simulink library "lib_HVESS"  (R2017a)
settings: Solver=VariableStepAuto  StartTime=0.0  StopTime=10.0  RelTol=1e-3
undefined symbols (not defined in the file): Atm_temp, bms_inletair_temp, bms_maxchargecurrent, bms_maxdischargecurrent, BMS_Notfallkuehlung, Cells, Chg, Em, ess, I_loss, mph2kph, R_0, R_1, SOC_bp, T_bp, tloop
libraries: fl_lib x13, simulink x9, nesl_utility x8, RollingAliveCounter x1
(part 2 of 2)

== stateflow chart lib_HVESS/ESS/Soft BMS/State Machine1/Startup_Shutdown_EPO_Sequence ==
  state BCM_ON
    state Default_Error_State
      en: BMS_Init_abgeschlossen=1;
      BMS_IstModus=5;
    state Standby
      en: BMS_Init_abgeschlossen=1;
      BMS_IstModus=0;
    state Normal_Driving
      en: NHM_BMS_Car_WakeUp=1;
      BMS_IstModus=1;
      BMS_Init_abgeschlossen=1;
      during: timer++;
    state Charging
      en:BMS_IstModus=4;
      BMS_Init_abgeschlossen =1;
      during: timer++;
    (default) -> Default_Error_State : [T_15&&T_30]
    Charging -> Default_Error_State [order 1] : [!T_30C]
    Normal_Driving -> Default_Error_State [order 1] : [!T_30C]
    (junction 134) -> Default_Error_State [order 2] : after(15, sec)[!T_30C]
    Default_Error_State -> Standby : [MO_BMS_Sollmodus==0&&...
        | Diag_Rq_Fktnl_Data_OBD==1]
        | %ErrorClear
    (junction 134) -> Standby [order 1] : [T_30C]
    Standby -> (junction 134) [order 3] : [!T_30C]
    Standby -> Charging [order 1] : [T_30C&&MO_BMS_Sollmodus==4]
        | %Standby>Charging
    Standby -> Normal_Driving [order 2] : [T_30C&&MO_BMS_Sollmodus==1]
        | {timer=0;}
        | %Standby>NormalDriving
    Normal_Driving -> Standby [order 2] : [T_30C&&MO_BMS_Sollmodus==0]
        | %NormalDriving>Standby
    Charging -> Standby [order 2] : [T_30C&&MO_BMS_Sollmodus==0]
        | %Charging>Standby
    Normal_Driving -> Charging [order 3] : [T_30C&&MO_BMS_Sollmodus==4] %NormalDriving>Charging
    Charging -> Normal_Driving [order 3] : [T_30C&&MO_BMS_Sollmodus==1] %Charging>NormalDriving
  state BCM_OFF
    state Prepare_to_Sleep
      en: NMH_BMS_Start_2=0;
      BMS_IstModus=5;
    state Ready_to_Sleep
      en: NMH_BMS_Normal_Mode_2=0;
      BMS_SleepInd=1;
      BMS_IstModus=5;
    state Bus_Sleep
      en: NMH_BMS_Start_1=0;
      BMS_SleepInd=1;
      BMS_IstModus=5;
    (default) -> Prepare_to_Sleep
    Prepare_to_Sleep -> Ready_to_Sleep : [timer>=0.05/tloop]
    Ready_to_Sleep -> Bus_Sleep : [timer>=0.05/tloop]
  note: !(veh_wake||chga_wake) || ...
      | !hsc_bcm_enable && !bcm_mainc_stat && bcm_cpwr_cmd]
  state EPO1
    BMS_Fehler_HS_offen=1;
    BMS_Fehler_HS_verschweisst =1;
    BMS_Fehler_HVBatt_Abschaltung=1;
    BMS_Fehler_HVBatt_Abschaltung_Anf=1;
    BMS_IstModus=5;
  state EPO
    BMS_Fehler_Notabschaltung_Crash=1;
    BMS_Fehler_Notabschaltung_Pilot=1;
    BMS_Fehler_Pilot=1;
    BMS_IstModus=5;
  (default) -> BCM_OFF
  BCM_OFF -> BCM_ON : [T_15&&T_30]
  BCM_ON -> BCM_OFF [order 1] : [T_15==0&&T_30==0]
  BCM_ON -> EPO1 [order 2] : [BattError|| SOC <=0.1]
  EPO1 -> BCM_OFF : [T_15==0&&T_30==0]
  EPO -> BCM_OFF : [T_15==0&&T_30==0]
  BCM_ON -> EPO [order 3] : after(2,sec)[CriticalBattError||MO_Fehler_Notentladung_Anf]
  data: timer local double; tloop parameter double; T_15 input double; T_30 input double; MO_BMS_Sollmodus input double; T_30C input double; BMS_Init_abgeschlossen output double; BMS_IstModus output double; BMS_Fehler_Pilot output double; NMH_Normal_Mode_1 output double; BMS_Fehler_HS_offen output double; BMS_Fehler_HS_verschweisst output double; NMH_BMS_Start_2 output double; NMH_BMS_Start_1 output double; BMS_Fehler_Notabschaltung_Crash output double; BMS_Fehler_Notabschaltung_Pilot output double; NHM_BMS_Car_WakeUp output double; BMS_SleepInd output double; NMH_BMS_Normal_Mode_2 output double; MO_Fehler_Notentladung_Anf input double; Diag_Rq_Fktnl_Data_OBD input boolean; BattError input boolean; CriticalBattError input boolean; BMS_Fehler_HVBatt_Abschaltung output double; BMS_Fehler_HVBatt_Abschaltung_Anf output double; SOC input double
